simulink model "Zencar_rpo_2020_IDENTIFICATION_simModel_flywheelSpring"  (R2020a)
settings: Solver=daessc  StartTime=0.0  StopTime=tsim  FixedStep=1e-3  MaxStep=1e-2  RelTol=1e-3
values from neighbouring files (symbols this model uses):
  A = [0 1 ; -k/I -b/I]    [Zencar_rpo_2020_IDENTIFICATION_runScript_flywheelSpring.m]    (also in Zencar_rpo_2020_IDENTIFICATION_spesession_flywheelSpring.mat = [0  1; -6.68094218415  -0.797644539615])
  Asys = [0 1 0 ; -k/I -b/I cfi/I ; 0 -cfi/L -R/L]    [Zencar_rpo_2020_IDENTIFICATION_feedForwardScript_flywheelSpring.m]    (also in Zencar_rpo_2020_IDENTIFICATION_runScript_flywheelSpring.m; Zencar_rpo_2020_IDENTIFICATION_spesession_flywheelSpring.mat = [0  1  0; -6.68094218415  -0.797644539615  25.5045739424; 0 )
  B = [0 ; 1/I]    [Zencar_rpo_2020_IDENTIFICATION_runScript_flywheelSpring.m]    (also in Zencar_rpo_2020_IDENTIFICATION_spesession_flywheelSpring.mat = [0 33.4140206005])
  Bsys = [0 ; 0 ; 1/L]    [Zencar_rpo_2020_IDENTIFICATION_feedForwardScript_flywheelSpring.m]    (also in Zencar_rpo_2020_IDENTIFICATION_runScript_flywheelSpring.m; Zencar_rpo_2020_IDENTIFICATION_spesession_flywheelSpring.mat = [0 0 166666.666667])
  C = [1 0]    [Zencar_rpo_2020_IDENTIFICATION_runScript_flywheelSpring.m]    (also in Zencar_rpo_2020_IDENTIFICATION_spesession_flywheelSpring.mat)
  Csys = [1 0 0;0 0 1]    [Zencar_rpo_2020_IDENTIFICATION_feedForwardScript_flywheelSpring.m]    (also in Zencar_rpo_2020_IDENTIFICATION_runScript_flywheelSpring.m; Zencar_rpo_2020_IDENTIFICATION_spesession_flywheelSpring.mat = [1  0  0; 0  0  1])
  D = [0]    [Zencar_rpo_2020_IDENTIFICATION_runScript_flywheelSpring.m]    (also in Zencar_rpo_2020_IDENTIFICATION_spesession_flywheelSpring.mat = 0)
  Dsys = [0;0]    [Zencar_rpo_2020_IDENTIFICATION_feedForwardScript_flywheelSpring.m]    (also in Zencar_rpo_2020_IDENTIFICATION_runScript_flywheelSpring.m; Zencar_rpo_2020_IDENTIFICATION_spesession_flywheelSpring.mat = [0 0])
  tchange = 12    [Zencar_rpo_2020_IDENTIFICATION_runScript_flywheelSpring.m]    (also in Zencar_rpo_2020_IDENTIFICATION_spesession_flywheelSpring.mat)
  U = 12    [Zencar_rpo_2020_IDENTIFICATION_runScript_flywheelSpring.m]    (also in Zencar_rpo_2020_IDENTIFICATION_spesession_flywheelSpring.mat)
settings Model: OrderedModelArguments=off  Creator=Honza  LastModifiedBy=Palo

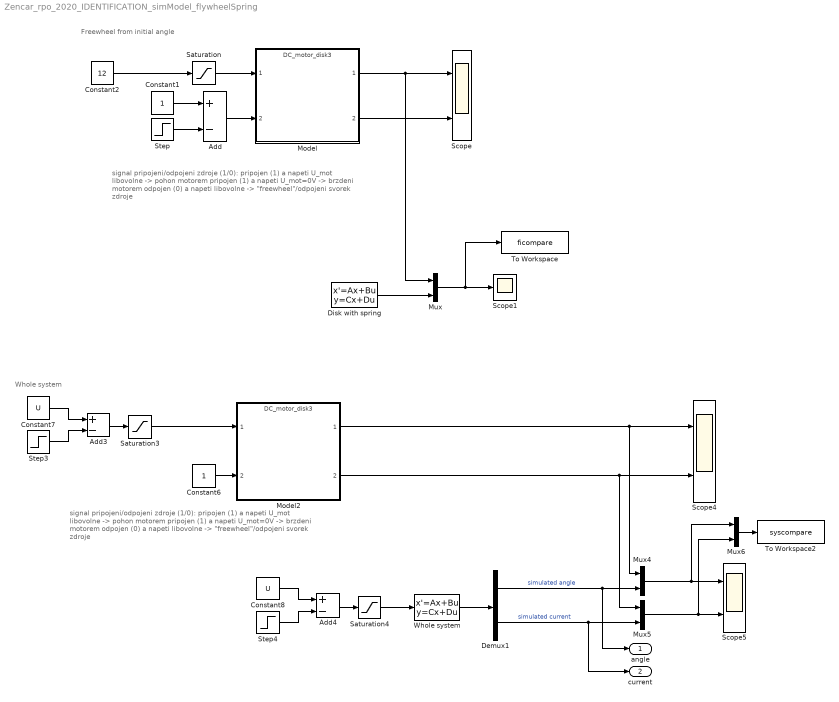
== system Zencar_rpo_2020_IDENTIFICATION_simModel_flywheelSpring ==
  note: Whole system
  note: Freewheel from initial angle
  note: signal pripojeni/odpojeni zdroje (1/0):
      |
      | pripojen (1) a napeti U_mot libovolne -> pohon motorem
      | pripojen (1) a napeti U_mot=0V -> brzdeni motorem
      | odpojen (0) a napeti libovolne -> "freewheel"/odpojeni svorek zdroje
  note: signal pripojeni/odpojeni zdroje (1/0):
      |
      | pripojen (1) a napeti U_mot libovolne -> pohon motorem
      | pripojen (1) a napeti U_mot=0V -> brzdeni motorem
      | odpojen (0) a napeti libovolne -> "freewheel"/odpojeni svorek zdroje
  Add : Sum  Inputs=+-
  Add3 : Sum  Inputs=+-
  Add4 : Sum  Inputs=+-
  Constant1 : Constant
  Constant2 : Constant  Value=12
  Constant6 : Constant
  Constant7 : Constant  Value=U
  Constant8 : Constant  Value=U
  Demux1 : Demux  Outputs=2
  Disk with spring : StateSpace  A=A  B=B  C=C  D=D  InitialCondition=[2.6789 0]
  Model : ModelReference  ModelNameDialog=DC_motor_disk3.slxp  ModelReferenceVersion=1.20  CopyOfModelProtected=on
  Model2 : ModelReference  ModelNameDialog=DC_motor_disk3.slxp  ModelReferenceVersion=1.20  CopyOfModelProtected=on
  Mux{,4..6} (4 alike) : Mux  Inputs=2
  Saturation : Saturate  UpperLimit=12  LowerLimit=-12
  Saturation3 : Saturate  UpperLimit=12  LowerLimit=-12
  Saturation4 : Saturate  UpperLimit=12  LowerLimit=-12
  Scope : Scope  NumInputPorts=2
  Scope1 : Scope
  Scope4 : Scope  NumInputPorts=2
  Scope5 : Scope  NumInputPorts=2
  Step : Step  Time=15  SampleTime=0
  Step3 : Step  Time=tchange  After=U  SampleTime=0
  Step4 : Step  Time=tchange  After=U  SampleTime=0
  To Workspace : ToWorkspace  VariableName=ficompare  SaveFormat=Structure With Time  SampleTime=-1
  To Workspace2 : ToWorkspace  VariableName=syscompare  SaveFormat=Structure With Time  SampleTime=-1
  Whole system : StateSpace  A=Asys  B=Bsys  C=Csys  D=Dsys  InitialCondition=[0 0 0]
  angle : Outport
  current : Outport  Port=2
  wires:
  Saturation/1 -> Model/1
  Mux/1 -> To Workspace/1, Scope1/1
  Constant1/1 -> Add/1
  Disk with spring/1 -> Mux/2
  Constant2/1 -> Saturation/1
  Model/2 -> Scope/2
  Step/1 -> Add/2
  Model/1 -> Mux/1, Scope/1
  Add/1 -> Model/2
  Demux1/1 -> angle/1, Mux4/2  "simulated angle"
  Demux1/2 -> current/1, Mux5/2  "simulated current"
  Mux6/1 -> To Workspace2/1
  Mux5/1 -> Scope5/2, Mux6/2
  Model2/1 -> Mux4/1, Scope4/1
  Add4/1 -> Saturation4/1
  Step4/1 -> Add4/2
  Constant8/1 -> Add4/1
  Constant7/1 -> Add3/1
  Saturation3/1 -> Model2/1
  Add3/1 -> Saturation3/1
  Mux4/1 -> Scope5/1, Mux6/1
  Step3/1 -> Add3/2
  Model2/2 -> Mux5/1, Scope4/2
  Constant6/1 -> Model2/2
  Whole system/1 -> Demux1/1
  Saturation4/1 -> Whole system/1
